simulink model "LugStateCtrl"  (R2018b)
settings: Solver=FixedStepDiscrete  StartTime=0.0  StopTime=10.0  FixedStep=0.01  RelTol=1e-3
settings Model: Creator=sn2xws  LastModifiedBy=sn2xws
settings DataIOCC: SaveFormat=StructureWithTime
settings OptimizationCC: DefaultParameterBehavior=Inlined  EnhancedBackFolding=on  PassReuseOutputArgsAs=Individual arguments  ZeroExternalMemoryAtStartup=off  ZeroInternalMemoryAtStartup=off  OptimizeBlockOrder=speed  DifferentSizesBufferReuse=on  OptimizationCustomize=off
settings DebuggingCC: ParameterTunabilityLossMsg=error
settings ModelReferenceCC: ModelReferenceNumInstancesAllowed=Single
settings SFSimCC: MATLABDynamicMemAlloc=off
settings RTWCC: SystemTargetFile=autosar.tlc  GenCodeOnly=on  TemplateMakefile=ert_default_tmf  Description=AUTOSAR  GenerateReport=on  IncludeHyperlinkInReport=on  LaunchReport=on  GenerateTraceInfo=on  GenerateTraceReport=on  GenerateTraceReportSl=on  GenerateTraceReportSf=on  GenerateTraceReportEml=on
settings CodeAppCC: ForceParamTrailComments=on  IgnoreCustomStorageClasses=off  OperatorAnnotations=on  SimulinkDataObjDesc=on  SFDataObjDesc=on  InsertBlockDesc=on
settings STFCustomTargetCC: TargetLangStandard=C99 (ISO)  MultiwordLength=256  ParMdlRefBuildCompliant=on  CompOptLevelCompliant=on  IncludeMdlTerminateFcn=off  CombineOutputUpdateFcns=on  SuppressErrorStatus=on  ERTCustomFileBanners=on  SupportNonFinite=off  SupportComplex=off  SupportContinuousTime=off  SupportNonInlinedSFcns=off  RemoveResetFunc=on  MATLABClassNameForMDSCustomization=Simulink.SoftwareTarget.ERTCustomization  AutosarCompliant=on  UseToolchainInfoCompliant=on  LookupTableObjectStructAxisOrder=2,1,3,4,...  LUTObjectStructOrderEvenSpacing=Size,Table,Breakpoints  SystemTargetFile=autosar.tlc
settings ERTTargetCC: TargetLangStandard=C99 (ISO)  ConcurrentExecutionCompliant=off  IncludeMdlTerminateFcn=off  SuppressErrorStatus=on  SupportNonFinite=off  SupportComplex=off  ModelStepFunctionPrototypeControlCompliant=off  CPPClassGenCompliant=off  AutosarCompliant=on  LookupTableObjectStructAxisOrder=2,1,3,4,...  LUTObjectStructOrderEvenSpacing=Size,Table,Breakpoints  InlinedParameterPlacement=NonHierarchical  ERTCustomFileTemplate=example_file_process.tlc

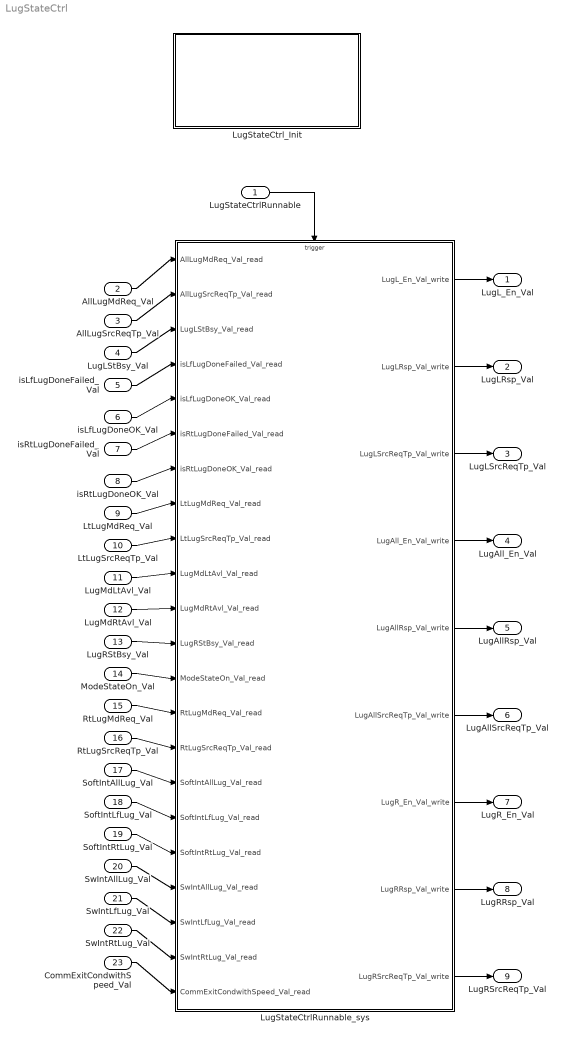
== system LugStateCtrl ==
  LugStateCtrlRunnable : Inport  SampleTime=0.01  OutputFunctionCall=on
  AllLugMdReq_Val : Inport  Port=2  OutDataTypeStr=boolean  PortDimensions=1
  AllLugSrcReqTp_Val : Inport  Port=3  OutDataTypeStr=Enum: SrcReqTp1  PortDimensions=1
  LugLStBsy_Val : Inport  Port=4  OutDataTypeStr=boolean  PortDimensions=1
  isLfLugDoneFailed_Val : Inport  Port=5  OutDataTypeStr=boolean  PortDimensions=1
  isLfLugDoneOK_Val : Inport  Port=6  OutDataTypeStr=boolean  PortDimensions=1
  isRtLugDoneFailed_Val : Inport  Port=7  OutDataTypeStr=boolean  PortDimensions=1
  isRtLugDoneOK_Val : Inport  Port=8  OutDataTypeStr=boolean  PortDimensions=1
  LtLugMdReq_Val : Inport  Port=9  OutDataTypeStr=boolean  PortDimensions=1
  LtLugSrcReqTp_Val : Inport  Port=10  OutDataTypeStr=Enum: SrcReqTp1  PortDimensions=1
  LugMdLtAvl_Val : Inport  Port=11  OutDataTypeStr=boolean  PortDimensions=1
  LugMdRtAvl_Val : Inport  Port=12  OutDataTypeStr=boolean  PortDimensions=1
  LugRStBsy_Val : Inport  Port=13  OutDataTypeStr=boolean  PortDimensions=1
  ModeStateOn_Val : Inport  Port=14  OutDataTypeStr=boolean  PortDimensions=1
  RtLugMdReq_Val : Inport  Port=15  OutDataTypeStr=boolean  PortDimensions=1
  RtLugSrcReqTp_Val : Inport  Port=16  OutDataTypeStr=Enum: SrcReqTp1  PortDimensions=1
  SoftIntAllLug_Val : Inport  Port=17  OutDataTypeStr=IntEnable  PortDimensions=1
  SoftIntLfLug_Val : Inport  Port=18  OutDataTypeStr=IntEnable  PortDimensions=1
  SoftIntRtLug_Val : Inport  Port=19  OutDataTypeStr=IntEnable  PortDimensions=1
  SwIntAllLug_Val : Inport  Port=20  OutDataTypeStr=IntEnable  PortDimensions=1
  SwIntLfLug_Val : Inport  Port=21  OutDataTypeStr=IntEnable  PortDimensions=1
  SwIntRtLug_Val : Inport  Port=22  OutDataTypeStr=IntEnable  PortDimensions=1
  CommExitCondwithSpeed_Val : Inport  Port=23  OutDataTypeStr=boolean  PortDimensions=1
  LugStateCtrlRunnable_sys : Subsystem
  LugStateCtrl_Init : Subsystem
  LugL_En_Val : Outport  OutDataTypeStr=boolean  PortDimensions=1
  LugLRsp_Val : Outport  Port=2  OutDataTypeStr=Enum: MdRspLocal1  PortDimensions=1
  LugLSrcReqTp_Val : Outport  Port=3  OutDataTypeStr=Enum: SrcReqTp1  PortDimensions=1
  LugAll_En_Val : Outport  Port=4  OutDataTypeStr=boolean  PortDimensions=1
  LugAllRsp_Val : Outport  Port=5  OutDataTypeStr=Enum: MdRspLocal1  PortDimensions=1
  LugAllSrcReqTp_Val : Outport  Port=6  OutDataTypeStr=Enum: SrcReqTp1  PortDimensions=1
  LugR_En_Val : Outport  Port=7  OutDataTypeStr=boolean  PortDimensions=1
  LugRRsp_Val : Outport  Port=8  OutDataTypeStr=Enum: MdRspLocal1  PortDimensions=1
  LugRSrcReqTp_Val : Outport  Port=9  OutDataTypeStr=Enum: SrcReqTp1  PortDimensions=1
  wires:
  AllLugMdReq_Val/1 -> LugStateCtrlRunnable_sys/1(AllLugMdReq_Val_read)
  AllLugSrcReqTp_Val/1 -> LugStateCtrlRunnable_sys/2(AllLugSrcReqTp_Val_read)
  LugLStBsy_Val/1 -> LugStateCtrlRunnable_sys/3(LugLStBsy_Val_read)
  isLfLugDoneFailed_Val/1 -> LugStateCtrlRunnable_sys/4(isLfLugDoneFailed_Val_read)
  isLfLugDoneOK_Val/1 -> LugStateCtrlRunnable_sys/5(isLfLugDoneOK_Val_read)
  isRtLugDoneFailed_Val/1 -> LugStateCtrlRunnable_sys/6(isRtLugDoneFailed_Val_read)
  isRtLugDoneOK_Val/1 -> LugStateCtrlRunnable_sys/7(isRtLugDoneOK_Val_read)
  LtLugMdReq_Val/1 -> LugStateCtrlRunnable_sys/8(LtLugMdReq_Val_read)
  LtLugSrcReqTp_Val/1 -> LugStateCtrlRunnable_sys/9(LtLugSrcReqTp_Val_read)
  LugMdLtAvl_Val/1 -> LugStateCtrlRunnable_sys/10(LugMdLtAvl_Val_read)
  LugMdRtAvl_Val/1 -> LugStateCtrlRunnable_sys/11(LugMdRtAvl_Val_read)
  LugRStBsy_Val/1 -> LugStateCtrlRunnable_sys/12(LugRStBsy_Val_read)
  ModeStateOn_Val/1 -> LugStateCtrlRunnable_sys/13(ModeStateOn_Val_read)
  RtLugMdReq_Val/1 -> LugStateCtrlRunnable_sys/14(RtLugMdReq_Val_read)
  RtLugSrcReqTp_Val/1 -> LugStateCtrlRunnable_sys/15(RtLugSrcReqTp_Val_read)
  SoftIntAllLug_Val/1 -> LugStateCtrlRunnable_sys/16(SoftIntAllLug_Val_read)
  SoftIntLfLug_Val/1 -> LugStateCtrlRunnable_sys/17(SoftIntLfLug_Val_read)
  SoftIntRtLug_Val/1 -> LugStateCtrlRunnable_sys/18(SoftIntRtLug_Val_read)
  SwIntAllLug_Val/1 -> LugStateCtrlRunnable_sys/19(SwIntAllLug_Val_read)
  SwIntLfLug_Val/1 -> LugStateCtrlRunnable_sys/20(SwIntLfLug_Val_read)
  SwIntRtLug_Val/1 -> LugStateCtrlRunnable_sys/21(SwIntRtLug_Val_read)
  LugStateCtrlRunnable_sys/1(LugL_En_Val_write) -> LugL_En_Val/1
  LugStateCtrlRunnable_sys/2(LugLRsp_Val_write) -> LugLRsp_Val/1
  LugStateCtrlRunnable_sys/3(LugLSrcReqTp_Val_write) -> LugLSrcReqTp_Val/1
  LugStateCtrlRunnable_sys/4(LugAll_En_Val_write) -> LugAll_En_Val/1
  LugStateCtrlRunnable_sys/5(LugAllRsp_Val_write) -> LugAllRsp_Val/1
  LugStateCtrlRunnable_sys/6(LugAllSrcReqTp_Val_write) -> LugAllSrcReqTp_Val/1
  LugStateCtrlRunnable_sys/7(LugR_En_Val_write) -> LugR_En_Val/1
  LugStateCtrlRunnable_sys/8(LugRRsp_Val_write) -> LugRRsp_Val/1
  LugStateCtrlRunnable_sys/9(LugRSrcReqTp_Val_write) -> LugRSrcReqTp_Val/1
  LugStateCtrlRunnable/1 -> LugStateCtrlRunnable_sys/Trigger
  CommExitCondwithSpeed_Val/1 -> LugStateCtrlRunnable_sys/22(CommExitCondwithSpeed_Val_read)

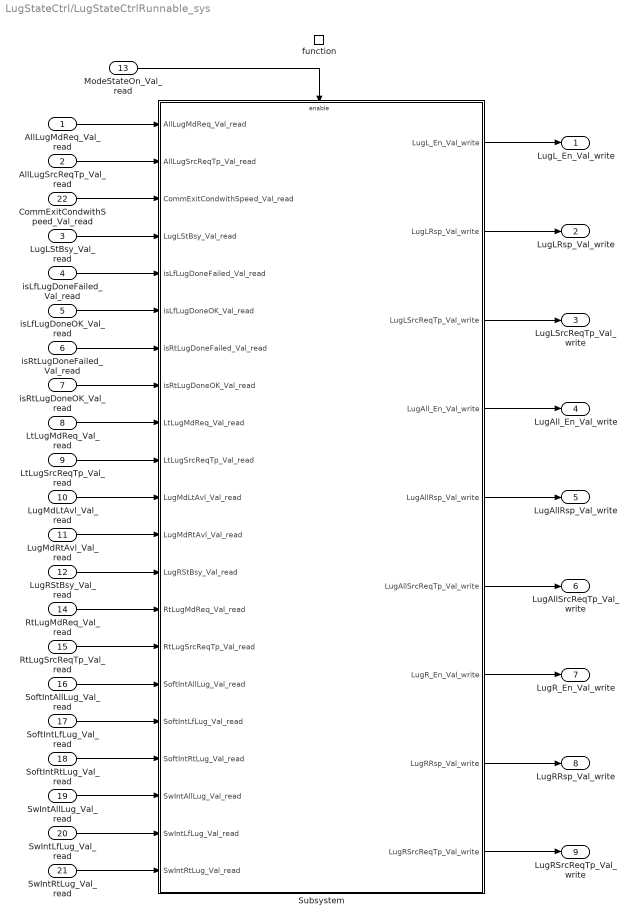
== system LugStateCtrl/LugStateCtrlRunnable_sys ==
  AllLugMdReq_Val_read : Inport
  AllLugSrcReqTp_Val_read : Inport  Port=2
  LugLStBsy_Val_read : Inport  Port=3
  isLfLugDoneFailed_Val_read : Inport  Port=4
  isLfLugDoneOK_Val_read : Inport  Port=5
  isRtLugDoneFailed_Val_read : Inport  Port=6
  isRtLugDoneOK_Val_read : Inport  Port=7
  LtLugMdReq_Val_read : Inport  Port=8
  LtLugSrcReqTp_Val_read : Inport  Port=9
  LugMdLtAvl_Val_read : Inport  Port=10
  LugMdRtAvl_Val_read : Inport  Port=11
  LugRStBsy_Val_read : Inport  Port=12
  ModeStateOn_Val_read : Inport  Port=13
  RtLugMdReq_Val_read : Inport  Port=14
  RtLugSrcReqTp_Val_read : Inport  Port=15
  SoftIntAllLug_Val_read : Inport  Port=16
  SoftIntLfLug_Val_read : Inport  Port=17
  SoftIntRtLug_Val_read : Inport  Port=18
  SwIntAllLug_Val_read : Inport  Port=19
  SwIntLfLug_Val_read : Inport  Port=20
  SwIntRtLug_Val_read : Inport  Port=21
  CommExitCondwithSpeed_Val_read : Inport  Port=22
  function : TriggerPort  TriggerType=function-call  VariantControl=(inherit)  SampleTimeType=periodic  SampleTime=-1
  Subsystem : Subsystem
  LugL_En_Val_write : Outport
      settings: EnsureOutportIsVirtual=on
  LugLRsp_Val_write : Outport  Port=2
      settings: EnsureOutportIsVirtual=on
  LugLSrcReqTp_Val_write : Outport  Port=3
      settings: EnsureOutportIsVirtual=on
  LugAll_En_Val_write : Outport  Port=4
      settings: EnsureOutportIsVirtual=on
  LugAllRsp_Val_write : Outport  Port=5
      settings: EnsureOutportIsVirtual=on
  LugAllSrcReqTp_Val_write : Outport  Port=6
      settings: EnsureOutportIsVirtual=on
  LugR_En_Val_write : Outport  Port=7
      settings: EnsureOutportIsVirtual=on
  LugRRsp_Val_write : Outport  Port=8
      settings: EnsureOutportIsVirtual=on
  LugRSrcReqTp_Val_write : Outport  Port=9
      settings: EnsureOutportIsVirtual=on
  wires:
  AllLugMdReq_Val_read/1 -> Subsystem/1(AllLugMdReq_Val_read)
  AllLugSrcReqTp_Val_read/1 -> Subsystem/2(AllLugSrcReqTp_Val_read)
  LugLStBsy_Val_read/1 -> Subsystem/4(LugLStBsy_Val_read)
  isLfLugDoneFailed_Val_read/1 -> Subsystem/5(isLfLugDoneFailed_Val_read)
  isLfLugDoneOK_Val_read/1 -> Subsystem/6(isLfLugDoneOK_Val_read)
  isRtLugDoneFailed_Val_read/1 -> Subsystem/7(isRtLugDoneFailed_Val_read)
  isRtLugDoneOK_Val_read/1 -> Subsystem/8(isRtLugDoneOK_Val_read)
  LtLugMdReq_Val_read/1 -> Subsystem/9(LtLugMdReq_Val_read)
  LtLugSrcReqTp_Val_read/1 -> Subsystem/10(LtLugSrcReqTp_Val_read)
  LugMdLtAvl_Val_read/1 -> Subsystem/11(LugMdLtAvl_Val_read)
  LugMdRtAvl_Val_read/1 -> Subsystem/12(LugMdRtAvl_Val_read)
  LugRStBsy_Val_read/1 -> Subsystem/13(LugRStBsy_Val_read)
  ModeStateOn_Val_read/1 -> Subsystem/Enable
  RtLugMdReq_Val_read/1 -> Subsystem/14(RtLugMdReq_Val_read)
  RtLugSrcReqTp_Val_read/1 -> Subsystem/15(RtLugSrcReqTp_Val_read)
  SoftIntAllLug_Val_read/1 -> Subsystem/16(SoftIntAllLug_Val_read)
  SoftIntLfLug_Val_read/1 -> Subsystem/17(SoftIntLfLug_Val_read)
  SoftIntRtLug_Val_read/1 -> Subsystem/18(SoftIntRtLug_Val_read)
  SwIntAllLug_Val_read/1 -> Subsystem/19(SwIntAllLug_Val_read)
  SwIntLfLug_Val_read/1 -> Subsystem/20(SwIntLfLug_Val_read)
  SwIntRtLug_Val_read/1 -> Subsystem/21(SwIntRtLug_Val_read)
  Subsystem/1(LugL_En_Val_write) -> LugL_En_Val_write/1
  Subsystem/2(LugLRsp_Val_write) -> LugLRsp_Val_write/1
  Subsystem/3(LugLSrcReqTp_Val_write) -> LugLSrcReqTp_Val_write/1
  Subsystem/4(LugAll_En_Val_write) -> LugAll_En_Val_write/1
  Subsystem/5(LugAllRsp_Val_write) -> LugAllRsp_Val_write/1
  Subsystem/6(LugAllSrcReqTp_Val_write) -> LugAllSrcReqTp_Val_write/1
  Subsystem/7(LugR_En_Val_write) -> LugR_En_Val_write/1
  Subsystem/8(LugRRsp_Val_write) -> LugRRsp_Val_write/1
  Subsystem/9(LugRSrcReqTp_Val_write) -> LugRSrcReqTp_Val_write/1
  CommExitCondwithSpeed_Val_read/1 -> Subsystem/3(CommExitCondwithSpeed_Val_read)

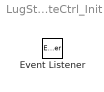
== system LugStateCtrl/LugStateCtrl_Init ==
  Event Listener : EventListener  EventName=reset

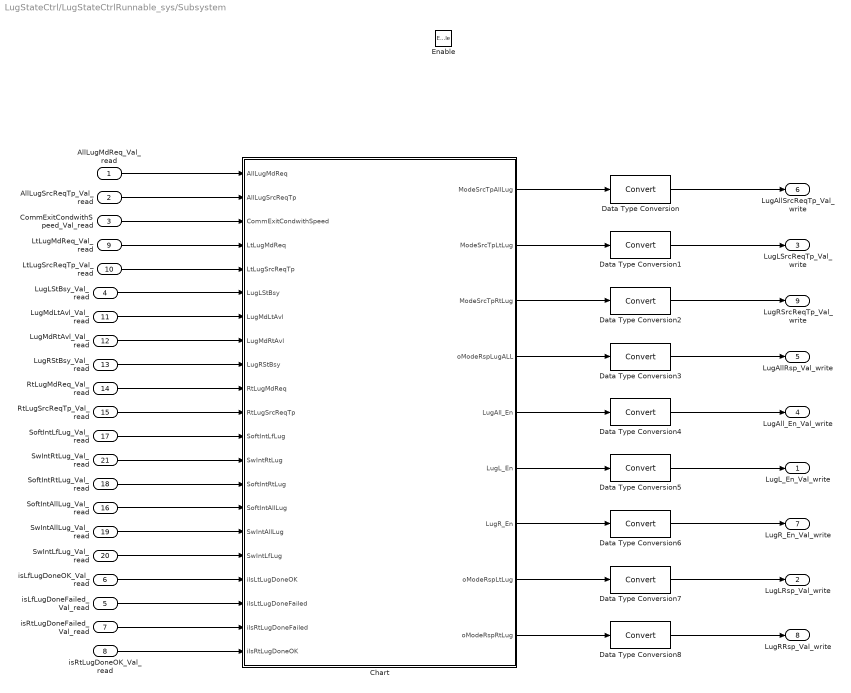
== system LugStateCtrl/LugStateCtrlRunnable_sys/Subsystem ==
  AllLugMdReq_Val_read : Inport
  AllLugSrcReqTp_Val_read : Inport  Port=2
  CommExitCondwithSpeed_Val_read : Inport  Port=3
  LugLStBsy_Val_read : Inport  Port=4
  isLfLugDoneFailed_Val_read : Inport  Port=5
  isLfLugDoneOK_Val_read : Inport  Port=6
  isRtLugDoneFailed_Val_read : Inport  Port=7
  isRtLugDoneOK_Val_read : Inport  Port=8
  LtLugMdReq_Val_read : Inport  Port=9
  LtLugSrcReqTp_Val_read : Inport  Port=10
  LugMdLtAvl_Val_read : Inport  Port=11
  LugMdRtAvl_Val_read : Inport  Port=12
  LugRStBsy_Val_read : Inport  Port=13
  RtLugMdReq_Val_read : Inport  Port=14
  RtLugSrcReqTp_Val_read : Inport  Port=15
  SoftIntAllLug_Val_read : Inport  Port=16
  SoftIntLfLug_Val_read : Inport  Port=17
  SoftIntRtLug_Val_read : Inport  Port=18
  SwIntAllLug_Val_read : Inport  Port=19
  SwIntLfLug_Val_read : Inport  Port=20
  SwIntRtLug_Val_read : Inport  Port=21
  Enable : EnablePort
  Chart : Stateflow chart  TreatAsAtomicUnit=on
  Data Type Conversion{,1..8} (9 alike) : DataTypeConversion
  LugL_En_Val_write : Outport
  LugLRsp_Val_write : Outport  Port=2
  LugLSrcReqTp_Val_write : Outport  Port=3
  LugAll_En_Val_write : Outport  Port=4
  LugAllRsp_Val_write : Outport  Port=5
  LugAllSrcReqTp_Val_write : Outport  Port=6
  LugR_En_Val_write : Outport  Port=7
  LugRRsp_Val_write : Outport  Port=8
  LugRSrcReqTp_Val_write : Outport  Port=9
  wires:
  AllLugMdReq_Val_read/1 -> Chart/1(AllLugMdReq)
  LugLStBsy_Val_read/1 -> Chart/6(LugLStBsy)
  LtLugSrcReqTp_Val_read/1 -> Chart/5(LtLugSrcReqTp)
  AllLugSrcReqTp_Val_read/1 -> Chart/2(AllLugSrcReqTp)
  Chart/6(LugL_En) -> Data Type Conversion5/1
  Chart/5(LugAll_En) -> Data Type Conversion4/1
  Chart/7(LugR_En) -> Data Type Conversion6/1
  Chart/3(ModeSrcTpRtLug) -> Data Type Conversion2/1
  Chart/2(ModeSrcTpLtLug) -> Data Type Conversion1/1
  Chart/1(ModeSrcTpAllLug) -> Data Type Conversion/1
  Chart/4(oModeRspLugALL) -> Data Type Conversion3/1
  Chart/8(oModeRspLtLug) -> Data Type Conversion7/1
  Chart/9(oModeRspRtLug) -> Data Type Conversion8/1
  LtLugMdReq_Val_read/1 -> Chart/4(LtLugMdReq)
  LugMdLtAvl_Val_read/1 -> Chart/7(LugMdLtAvl)
  LugMdRtAvl_Val_read/1 -> Chart/8(LugMdRtAvl)
  LugRStBsy_Val_read/1 -> Chart/9(LugRStBsy)
  RtLugMdReq_Val_read/1 -> Chart/10(RtLugMdReq)
  RtLugSrcReqTp_Val_read/1 -> Chart/11(RtLugSrcReqTp)
  isLfLugDoneFailed_Val_read/1 -> Chart/19(iIsLtLugDoneFailed)
  isLfLugDoneOK_Val_read/1 -> Chart/18(iIsLtLugDoneOK)
  isRtLugDoneFailed_Val_read/1 -> Chart/20(iIsRtLugDoneFailed)
  isRtLugDoneOK_Val_read/1 -> Chart/21(iIsRtLugDoneOK)
  SoftIntAllLug_Val_read/1 -> Chart/15(SoftIntAllLug)
  SoftIntLfLug_Val_read/1 -> Chart/12(SoftIntLfLug)
  SoftIntRtLug_Val_read/1 -> Chart/14(SoftIntRtLug)
  SwIntAllLug_Val_read/1 -> Chart/16(SwIntAllLug)
  SwIntLfLug_Val_read/1 -> Chart/17(SwIntLfLug)
  SwIntRtLug_Val_read/1 -> Chart/13(SwIntRtLug)
  CommExitCondwithSpeed_Val_read/1 -> Chart/3(CommExitCondwithSpeed)
  Data Type Conversion/1 -> LugAllSrcReqTp_Val_write/1
  Data Type Conversion1/1 -> LugLSrcReqTp_Val_write/1
  Data Type Conversion2/1 -> LugRSrcReqTp_Val_write/1
  Data Type Conversion3/1 -> LugAllRsp_Val_write/1
  Data Type Conversion4/1 -> LugAll_En_Val_write/1
  Data Type Conversion5/1 -> LugL_En_Val_write/1
  Data Type Conversion6/1 -> LugR_En_Val_write/1
  Data Type Conversion7/1 -> LugLRsp_Val_write/1
  Data Type Conversion8/1 -> LugRRsp_Val_write/1

== stateflow chart LugStateCtrl/LugStateCtrlRunnable_sys/Subsystem/Chart ==
  state ChkLugAll [function]
    (default) -> (junction 2)
    (junction 2) -> (junction 3) [order 1] : [LugAll_En ==1&&LugL_En==0&&LugR_En==0]
    (junction 3) -> (junction 4) [order 1] : [LugMdLtAvl ==LugMdRtAvl && oModeRspLtLug ==oModeRspRtLug]
    (junction 2) -> (junction 5) [order 2]
    (junction 3) -> (junction 6) [order 2] : {
        | LugAll_En=0;
        | oModeRspLugALL =MdRsp_RecallUnsuccessfully_Error;
        | ModeSrcTpAllLug=SrcReqTp1.SrcReqTp_None;
        | }
    (junction 4) -> (junction 7) : {
        | LugAll_En = 0;
        | oModeRspLugALL =oModeRspLtLug;
        | ModeSrcTpAllLug =  SrcReqTp1.SrcReqTp_None;
        | }
    (junction 6) -> (junction 5)
    (junction 7) -> (junction 6)
  state LugStateCtrl
    state LugL [parallel]
      settings: executionOrder=1
      state LugLIlde
        en:LugL_En =0;
        en:ModeSrcTpLtLug =SrcReqTp1.SrcReqTp_None;
        en:ChkLugAll();
      state LugLtOngoing
        en:LugL_En =1;
        en:ModeSrcTpAllLug = AllLugSrcReqTp;
        en:oModeRspLtLug = MdRsp_RecallOngoing;
      (default) -> LugLIlde
      LugLIlde -> LugLtOngoing [order 1] : [(AllLugMdReq)&&LugLStBsy ==0&&LugMdLtAvl ==1]
          | {LugAll_En=1;oModeRspLugALL=MdRsp_RecallOngoing;ModeSrcTpLtLug = AllLugSrcReqTp;}
      LugLIlde -> LugLtOngoing [order 2] : [(LtLugMdReq)&&LugLStBsy ==0]{ModeSrcTpLtLug = LtLugSrcReqTp;}
      LugLtOngoing -> LugLIlde [order 1] : [hasChangedTo(SoftIntLfLug,true)...
          | ||(hasChangedTo(SoftIntAllLug,true)&&LugAll_En)]
          | {oModeRspLtLug = MdRsp_RecallUnsuccessfully_LocalInterrupt;}
      LugLtOngoing -> LugLIlde [order 2] : [hasChangedTo(SwIntLfLug,true)...
          | ||(hasChangedTo(SwIntAllLug,true)&&LugAll_En)]
          | {oModeRspLtLug = MdRsp_RecallUnsuccessfully_LocalInterrupt;}
      LugLtOngoing -> LugLIlde [order 3] : [hasChangedTo(iIsLtLugDoneOK,true) ]
          | {oModeRspLtLug = MdRsp_RecallSuccessfully;} /*<REQ_MSM_420>*/
      LugLtOngoing -> LugLIlde [order 4] : [CommExitCondwithSpeed]{oModeRspLtLug = MdRsp_RecallUnsuccessfully_Error;} /*<REQ_MSM_435>*/
      LugLtOngoing -> LugLIlde [order 5] : [hasChangedTo(iIsLtLugDoneFailed,true)]
          | {oModeRspLtLug = MdRsp_RecallUnsuccessfully_Error;}/*<REQ_MSM_420>*/
    state LugR [parallel]
      settings: executionOrder=2
      state LugRtOngoing
        en:LugR_En = 1;
        en:ModeSrcTpAllLug = AllLugSrcReqTp;
        en:oModeRspRtLug = MdRsp_RecallOngoing;
      state LugRIdle
        en:LugR_En =0;
        en:ModeSrcTpRtLug =SrcReqTp1.SrcReqTp_None;
        en:ChkLugAll();
      (default) -> LugRIdle
      LugRIdle -> LugRtOngoing [order 1] : [(AllLugMdReq)&&LugRStBsy ==0&&LugMdRtAvl==1]
          | {LugAll_En=1;oModeRspLugALL=MdRsp_RecallOngoing;ModeSrcTpRtLug = AllLugSrcReqTp;}
      LugRIdle -> LugRtOngoing [order 2] : [(RtLugMdReq)&&LugRStBsy ==0]{ModeSrcTpRtLug = RtLugSrcReqTp;}
      LugRtOngoing -> LugRIdle [order 1] : [hasChangedTo(SoftIntRtLug,true)...
          | ||(hasChangedTo(SoftIntAllLug,true)&&LugAll_En)]{oModeRspRtLug = MdRsp_RecallUnsuccessfully_LocalInterrupt;}
      LugRtOngoing -> LugRIdle [order 2] : [hasChangedTo(SwIntRtLug,true)...
          | ||(hasChangedTo(SwIntAllLug,true)&&LugAll_En)]{oModeRspRtLug = MdRsp_RecallUnsuccessfully_LocalInterrupt; }
      LugRtOngoing -> LugRIdle [order 3] : [hasChangedTo(iIsRtLugDoneOK,true)]{oModeRspRtLug = MdRsp_RecallSuccessfully;}
      LugRtOngoing -> LugRIdle [order 4] : [CommExitCondwithSpeed]{oModeRspRtLug = MdRsp_RecallUnsuccessfully_Error;}
      LugRtOngoing -> LugRIdle [order 5] : [hasChangedTo(iIsRtLugDoneFailed,true)]{oModeRspRtLug = MdRsp_RecallUnsuccessfully_Error;}
  (default) -> LugStateCtrl
  data: AllLugMdReq input; AllLugSrcReqTp input; CommExitCondwithSpeed input; LtLugMdReq input; LtLugSrcReqTp input; LugLStBsy input; LugMdLtAvl input; LugMdRtAvl input; LugRStBsy input; RtLugMdReq input; RtLugSrcReqTp input; ModeSrcTpAllLug output Enum: SrcReqTp1; ModeSrcTpLtLug output Enum: SrcReqTp1; ModeSrcTpRtLug output Enum: SrcReqTp1; oModeRspLugALL output Enum: MdRspLocal1; LugAll_En output boolean; LugL_En output boolean; LugR_En output boolean; oModeRspLtLug output Enum: MdRspLocal1; oModeRspRtLug output Enum: MdRspLocal1; SoftIntLfLug input; SwIntRtLug input; SoftIntRtLug input; SoftIntAllLug input; SwIntAllLug input; SwIntLfLug input; iIsLtLugDoneOK input; iIsLtLugDoneFailed input; iIsRtLugDoneFailed input; iIsRtLugDoneOK input
